simulink model "Circuito_RL_Simulink"  (R2023b)
settings: Solver=VariableStepAuto  StartTime=0.0  StopTime=0.00005  RelTol=1e-3
settings Model: Creator=tomas  LastModifiedBy=tomas

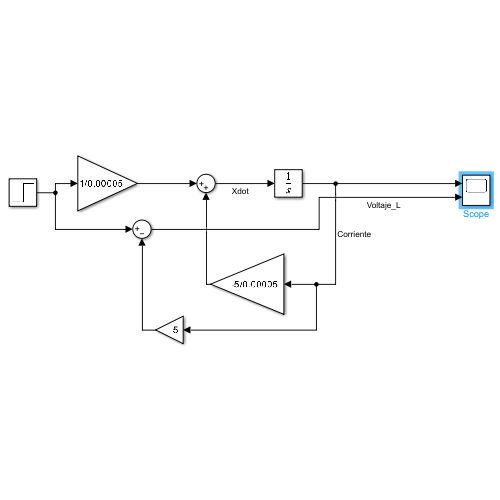
[thumbnail: Simulink's stored preview of the top-level diagram]
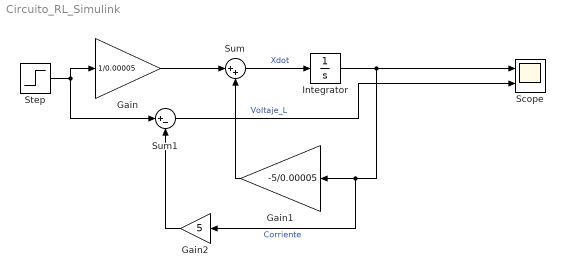
== system Circuito_RL_Simulink ==
  Gain : Gain  Gain=1/0.00005
  Gain1 : Gain  Gain=-5/0.00005
  Gain2 : Gain  Gain=5
  Integrator : Integrator
  Scope : Scope  NumInputPorts=2
  Step : Step  Time=0  After=10  SampleTime=0
  Sum : Sum  Inputs=|++
  Sum1 : Sum  Inputs=|+-
  wires:
  Sum/1 -> Integrator/1  "Xdot"
  Integrator/1 -> Gain2/1, Gain1/1, Scope/1  "Corriente"
  Gain1/1 -> Sum/2
  Gain/1 -> Sum/1
  Step/1 -> Sum1/1, Gain/1
  Gain2/1 -> Sum1/2
  Sum1/1 -> Scope/2  "Voltaje_L"
